simulink model "Q9_Simulink"  (R2019a)
settings: Solver=VariableStepAuto  StartTime=0.0  StopTime=simTime  RelTol=1e-8
values from neighbouring files (symbols this model uses):
  atan_scale = 100    [Q6.mat]    (also in Q8.mat)
  b_1 = 0.0029    [Q6.mat]    (also in Q8.mat)
  b_2 = 0.0002    [Q6.mat]    (also in Q8.mat)
  b_3 = 0.00015    [Q6.mat]    (also in Q8.mat)
  C = [1 0 0 0 0 0 0 1 0 0 0 0 ... (18 elements, 3x6)]    [Q6.mat]    (also in Q8.mat)
  C_ref = [1.22433209487 0.111020135599 0.137798657392 0.044869064232 0.221712033644 0.0486858100967]    [Q8.mat]
  F = [0.991402974605 -4.28040333336 0.0119339997062 5.93452176144 2.30402133564e-05 0.0230057113747 0.0039792647266 0.986787027522 1.59283068262e-05 0.0119155228703 1.84337564103e-08 2.30188301989e-05 ... (36 elements, 6x6)]    [Q8.mat]
  f_m = 0.00325471482319    [Q6.mat]
  f_m_time = 5    [Q6.mat]
  G = [0.00319046326914 1.59170589064 6.37978954487e-06 0.00637132273049 4.91886463074e-09 7.3735025641e-06]    [Q8.mat]
  h_sol = 17.717102911    [Q6.mat]
  J_1 = 0.0025    [Q6.mat]    (also in Q8.mat)
  J_2 = 0.0018    [Q6.mat]    (also in Q8.mat)
  J_3 = 0.0018    [Q6.mat]    (also in Q8.mat)
  k_1 = 2.7    [Q6.mat]    (also in Q8.mat)
  k_2 = 2.6    [Q6.mat]    (also in Q8.mat)
  Kc = [0.596249461469 0.0540667816687 0.0671079159043 0.0218512244326 0.10797371172 0.0237099788309]    [Q8.mat]
  mu_0 = 0    [Q6.mat]
  mu_1_sol = -0.0172499885629    [Q6.mat]
  T_Cm = 0.0969711017207    [Q6.mat]    (also in Q8.mat)
  T_Cp = 0.0714454263135    [Q6.mat]    (also in Q8.mat)
  T_s = 0.004    [Q6.mat]
  theta_3_ref = 1.57079632679    [Q8.mat]
  Ts = 0.004    [Q8.mat]
  var_r0 = 0.0043741038014    [Q6.mat]
  w_th = 0.75    [Q6.mat]    (also in Q8.mat)
  x_0 = [0 0 0 0 0 0]    [Q6.mat]
undefined symbols (not defined in the file or in its folder): C_f, C_V_d, G_V, G_y1_d, G_y2_d, G_y3_d, L_d, L_V_d, P_V_d, sigma_meas
settings Model: Creator=dimpa  LastModifiedBy=Ian
settings DataIOCC: ReturnWorkspaceOutputs=off
settings DebuggingCC: ArithmeticOperatorsInVariantConditions=warning
settings SFSimCC: SimUseLocalCustomCode=off
settings RTWCC: RTWUseLocalCustomCode=off

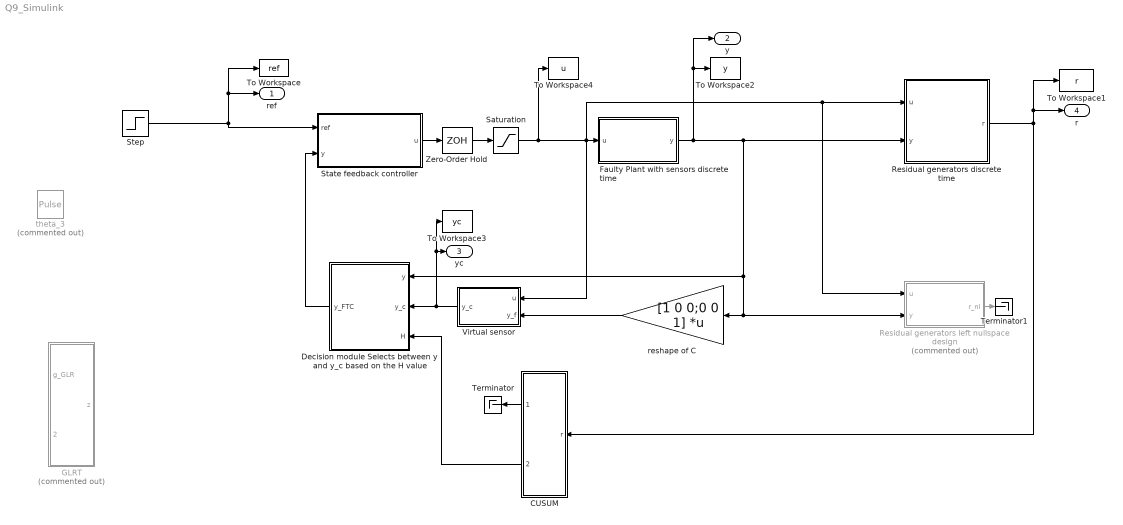
== system Q9_Simulink ==
  CUSUM : Subsystem
  Decision module Selects between y and y_c based on the H value : Subsystem
  Faulty Plant with sensors discrete time : Subsystem
  GLRT : Subsystem  Commented=on
  Residual generators discrete time : Subsystem
  Residual generators left nullspace design : Subsystem  Commented=on
  Saturation : Saturate  UpperLimit=2  LowerLimit=-2
  State feedback controller : Subsystem
  Step : Step  Time=15  After=theta_3_ref  SampleTime=0
  Terminator : Terminator
  Terminator1 : Terminator
  To Workspace : ToWorkspace  VariableName=ref  SaveFormat=Structure With Time  SampleTime=-1
  To Workspace1 : ToWorkspace  VariableName=r  SaveFormat=Structure With Time  SampleTime=-1
  To Workspace2 : ToWorkspace  VariableName=y  SaveFormat=Structure With Time  SampleTime=-1
  To Workspace3 : ToWorkspace  VariableName=yc  SaveFormat=Structure With Time  SampleTime=-1
  To Workspace4 : ToWorkspace  VariableName=u  SaveFormat=Structure With Time  SampleTime=-1
  Virtual sensor : Subsystem
  Zero-Order Hold : ZeroOrderHold  SampleTime=T_s
  reshape of C : Gain  Gain=[1 0 0;0 0 1]  Multiplication=Matrix(K*u) (u vector)
  theta_3 : DiscretePulseGenerator  Commented=on  PulseType=Time based  Amplitude=theta_3_ref  Period=30  PulseWidth=50
  ref : Outport  VectorParamsAs1DForOutWhenUnconnected=on
  y : Outport  Port=2  VectorParamsAs1DForOutWhenUnconnected=on
  yc : Outport  Port=3  VectorParamsAs1DForOutWhenUnconnected=on
  r : Outport  Port=4  VectorParamsAs1DForOutWhenUnconnected=on
  wires:
  State feedback controller/1(u) -> Zero-Order Hold/1
  Saturation/1 -> To Workspace4/1, Virtual sensor/1(u), Residual generators discrete time/1(u), Residual generators left nullspace design/1(u), Faulty Plant with sensors discrete time/1(u)
  Faulty Plant with sensors discrete time/1(y) -> y/1, To Workspace2/1, Residual generators discrete time/2(y), Decision module Selects between y and y_c based on the H value/1(y), reshape of C/1, Residual generators left nullspace design/2(y)
  Step/1 -> State feedback controller/1(ref), ref/1, To Workspace/1
  Virtual sensor/1(y_c) -> yc/1, To Workspace3/1, Decision module Selects between y and y_c based on the H value/2(y_c)
  reshape of C/1 -> Virtual sensor/2(y_f)
  Zero-Order Hold/1 -> Saturation/1
  CUSUM/2(H_CUSUM) -> Decision module Selects between y and y_c based on the H value/3(H)
  CUSUM/1(g_CUSUM) -> Terminator/1
  Residual generators left nullspace design/1(r_nl) -> Terminator1/1
  Residual generators discrete time/1(r) -> r/1, To Workspace1/1, CUSUM/1(r)
  Decision module Selects between y and y_c based on the H value/1(y_FTC) -> State feedback controller/2(y)

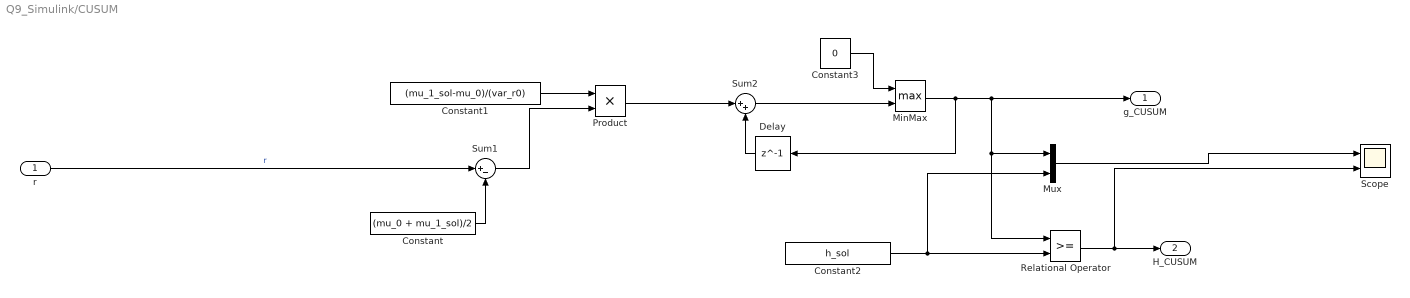
== system Q9_Simulink/CUSUM ==
  r : Inport
  Constant : Constant  Value=(mu_0 + mu_1_sol)/2
  Constant1 : Constant  Value=(mu_1_sol-mu_0)/(var_r0)
  Constant2 : Constant  Value=h_sol  VectorParams1D=off
  Constant3 : Constant  Value=0
  Delay : Delay  DelayLength=1  SampleTime=0.004
  MinMax : MinMax  Function=max  Inputs=2
  Mux : Mux  Inputs=2
  Product : Product
  Relational Operator : RelationalOperator  OutDataTypeStr=boolean  RndMeth=Simplest
  Scope : Scope  NumInputPorts=2
  Sum1 : Sum  Inputs=|+-
  Sum2 : Sum  Inputs=|++
  g_CUSUM : Outport
  H_CUSUM : Outport  Port=2
  wires:
  MinMax/1 -> Delay/1, g_CUSUM/1, Mux/1, Relational Operator/1
  Mux/1 -> Scope/1
  Delay/1 -> Sum2/2
  Constant2/1 -> Mux/2, Relational Operator/2
  Product/1 -> Sum2/1
  Constant3/1 -> MinMax/1
  Constant/1 -> Sum1/2
  Constant1/1 -> Product/1
  Sum1/1 -> Product/2
  Relational Operator/1 -> H_CUSUM/1, Scope/2
  Sum2/1 -> MinMax/2
  r/1 -> Sum1/1  "r"

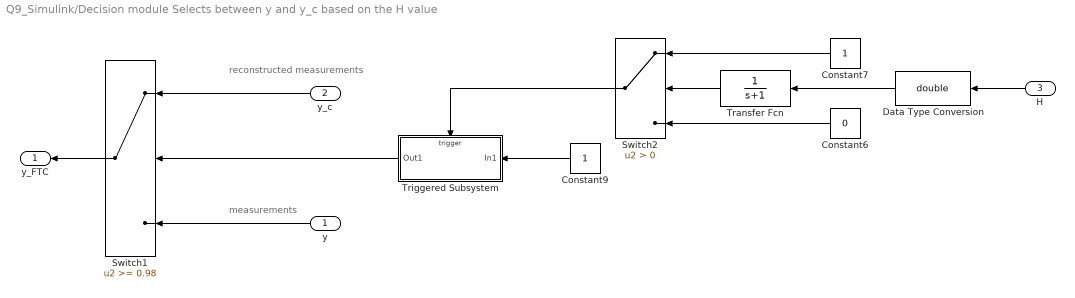
== system Q9_Simulink/Decision module Selects between y and y_c based on the H value ==
  note: measurements
  note: reconstructed
      | measurements
  y : Inport
  y_c : Inport  Port=2
  H : Inport  Port=3
  Constant6 : Constant  Value=0
  Constant7 : Constant
  Constant9 : Constant
  Data Type Conversion : DataTypeConversion  OutDataTypeStr=double
  Switch1 : Switch  Threshold=0.98
  Switch2 : Switch  Criteria=u2 > Threshold
  Transfer Fcn : TransferFcn  Denominator=[1 1]
  Triggered Subsystem : Subsystem  TreatAsAtomicUnit=on
  y_FTC : Outport
  wires:
  Switch1/1 -> y_FTC/1
  Constant6/1 -> Switch2/3
  Constant9/1 -> Triggered Subsystem/1(In1)
  Switch2/1 -> Triggered Subsystem/Trigger
  Constant7/1 -> Switch2/1
  Transfer Fcn/1 -> Switch2/2
  y/1 -> Switch1/3
  y_c/1 -> Switch1/1
  H/1 -> Data Type Conversion/1
  Triggered Subsystem/1(Out1) -> Switch1/2
  Data Type Conversion/1 -> Transfer Fcn/1

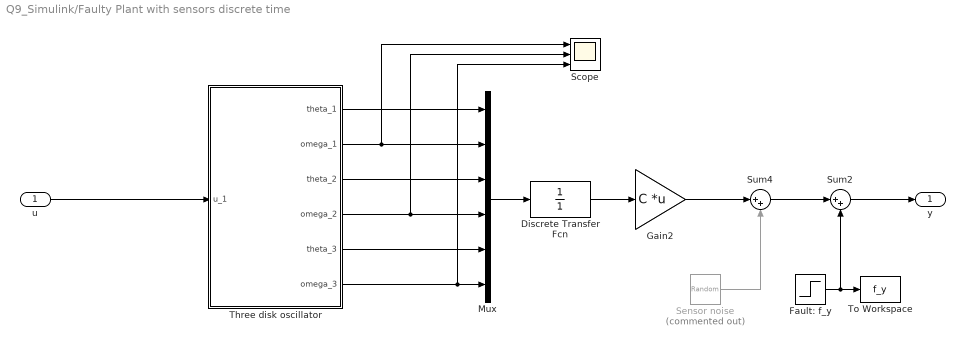
== system Q9_Simulink/Faulty Plant with sensors discrete time ==
  u : Inport
  Discrete Transfer Fcn : DiscreteTransferFcn  Denominator=[1]  SampleTime=T_s
  Fault: f_y : Step  Time=f_m_time  Before=[0;0;0]  After=f_m  SampleTime=0
  Gain2 : Gain  Gain=C  Multiplication=Matrix(K*u) (u vector)
  Mux : Mux  Inputs=6
  Scope : Scope  NumInputPorts=3
  Sensor noise : RandomNumber  Commented=on  Mean=zeros(3,1)  Variance=sigma_meas  SampleTime=T_s
  Sum2 : Sum  Inputs=|++
  Sum4 : Sum  Inputs=|++
  Three disk oscillator : Subsystem
  To Workspace : ToWorkspace  VariableName=f_y  SaveFormat=Structure With Time  SampleTime=-1
  y : Outport
  wires:
  u/1 -> Three disk oscillator/1(u_1)
  Three disk oscillator/2(omega_1) -> Scope/1, Mux/2
  Three disk oscillator/1(theta_1) -> Mux/1
  Mux/1 -> Discrete Transfer Fcn/1
  Three disk oscillator/4(omega_2) -> Scope/2, Mux/4
  Three disk oscillator/3(theta_2) -> Mux/3
  Discrete Transfer Fcn/1 -> Gain2/1
  Gain2/1 -> Sum4/1
  Sum2/1 -> y/1
  Sensor noise/1 -> Sum4/2
  Three disk oscillator/6(omega_3) -> Scope/3, Mux/6
  Three disk oscillator/5(theta_3) -> Mux/5
  Sum4/1 -> Sum2/1
  Fault: f_y/1 -> To Workspace/1, Sum2/2

== system Q9_Simulink/GLRT ==
  z : Inport
  g_GLR : Outport
  H_GLR : Outport  Port=2

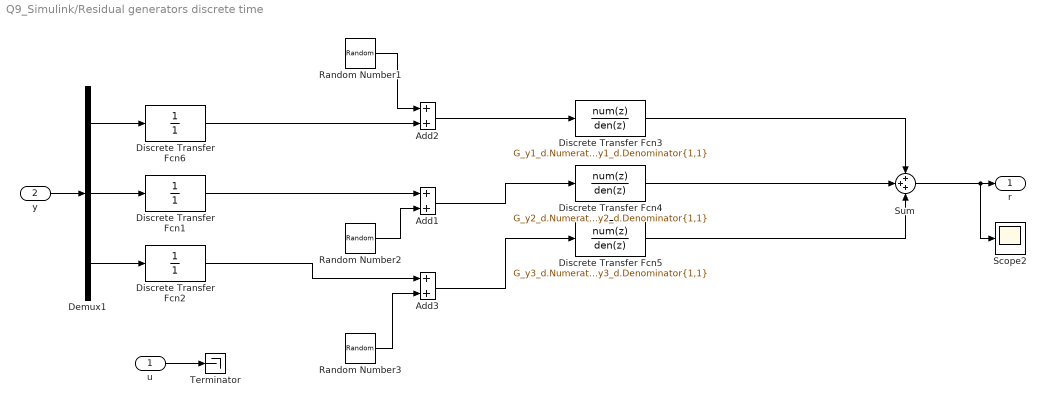
== system Q9_Simulink/Residual generators discrete time ==
  u : Inport
  y : Inport  Port=2
  Add1 : Sum
  Add2 : Sum
  Add3 : Sum
  Demux1 : Demux  Outputs=3
  Discrete Transfer Fcn1 : DiscreteTransferFcn  Denominator=[1]  SampleTime=0.004
  Discrete Transfer Fcn2 : DiscreteTransferFcn  Denominator=[1]  SampleTime=0.004
  Discrete Transfer Fcn3 : DiscreteTransferFcn  Numerator=G_y1_d.Numerator{1,1}  Denominator=G_y1_d.Denominator{1,1}
  Discrete Transfer Fcn4 : DiscreteTransferFcn  Numerator=G_y2_d.Numerator{1,1}  Denominator=G_y2_d.Denominator{1,1}
  Discrete Transfer Fcn5 : DiscreteTransferFcn  Numerator=G_y3_d.Numerator{1,1}  Denominator=G_y3_d.Denominator{1,1}
  Discrete Transfer Fcn6 : DiscreteTransferFcn  Denominator=[1]  SampleTime=0.004
  Random Number1 : RandomNumber  Variance=0.01^2  Seed=124234  SampleTime=T_s
  Random Number2 : RandomNumber  Variance=0.01^2  Seed=245364  SampleTime=T_s
  Random Number3 : RandomNumber  Variance=0.01^2  Seed=1465  SampleTime=T_s
  Scope2 : Scope
  Sum : Sum  Inputs=+++
  Terminator : Terminator
  r : Outport
  wires:
  u/1 -> Terminator/1
  Discrete Transfer Fcn4/1 -> Sum/2
  Sum/1 -> r/1, Scope2/1
  Add1/1 -> Discrete Transfer Fcn4/1
  Discrete Transfer Fcn5/1 -> Sum/3
  Random Number2/1 -> Add1/2
  Discrete Transfer Fcn3/1 -> Sum/1
  Random Number3/1 -> Add3/2
  Discrete Transfer Fcn2/1 -> Add3/1
  Add3/1 -> Discrete Transfer Fcn5/1
  y/1 -> Demux1/1
  Demux1/1 -> Discrete Transfer Fcn6/1
  Discrete Transfer Fcn6/1 -> Add2/2
  Random Number1/1 -> Add2/1
  Add2/1 -> Discrete Transfer Fcn3/1
  Demux1/2 -> Discrete Transfer Fcn1/1
  Discrete Transfer Fcn1/1 -> Add1/1
  Demux1/3 -> Discrete Transfer Fcn2/1

== system Q9_Simulink/Residual generators left nullspace design ==
  u : Inport
  y : Inport  Port=2
  r_nl : Outport

== system Q9_Simulink/State feedback controller ==
  ref : Inport
  y : Inport  Port=2
  State feedback with linear observer : Subsystem
  u : Outport
  wires:
  ref/1 -> State feedback with linear observer/1(ref)
  y/1 -> State feedback with linear observer/2(y)
  State feedback with linear observer/1(u) -> u/1

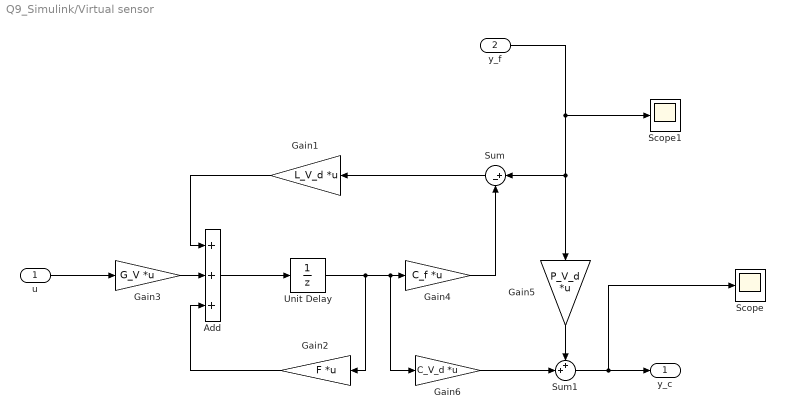
== system Q9_Simulink/Virtual sensor ==
  u : Inport
  y_f : Inport  Port=2
  Add : Sum  Inputs=+++
  Gain1 : Gain  Gain=L_V_d  Multiplication=Matrix(K*u)
  Gain2 : Gain  Gain=F  Multiplication=Matrix(K*u)
  Gain3 : Gain  Gain=G_V  Multiplication=Matrix(K*u)
  Gain4 : Gain  Gain=C_f  Multiplication=Matrix(K*u)
  Gain5 : Gain  Gain=P_V_d  Multiplication=Matrix(K*u)
  Gain6 : Gain  Gain=C_V_d  Multiplication=Matrix(K*u)
  Scope : Scope
  Scope1 : Scope
  Sum : Sum  Inputs=|+-
  Sum1 : Sum  Inputs=++|
  Unit Delay : UnitDelay  SampleTime=Ts  HasFrameUpgradeWarning=on
  y_c : Outport
  wires:
  u/1 -> Gain3/1
  Gain3/1 -> Add/2
  Gain1/1 -> Add/1
  Gain2/1 -> Add/3
  Add/1 -> Unit Delay/1
  Unit Delay/1 -> Gain6/1, Gain4/1, Gain2/1
  Sum/1 -> Gain1/1
  Gain4/1 -> Sum/2
  y_f/1 -> Scope1/1, Sum/1, Gain5/1
  Gain6/1 -> Sum1/2
  Gain5/1 -> Sum1/1
  Sum1/1 -> Scope/1, y_c/1

== system Q9_Simulink/Decision module Selects between y and y_c based on the H value/Triggered Subsystem ==
  In1 : Inport
  Trigger : TriggerPort  VariantControl=Variant
  Out1 : Outport
  wires:
  In1/1 -> Out1/1

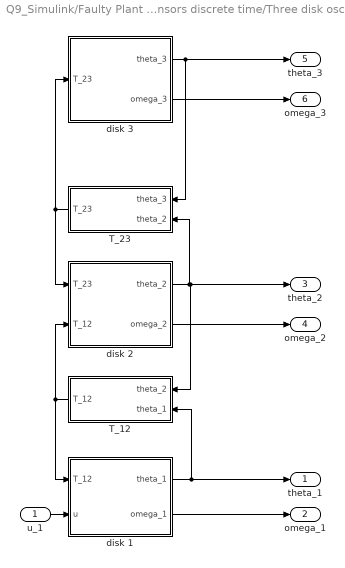
== system Q9_Simulink/Faulty Plant with sensors discrete time/Three disk oscillator ==
  u_1 : Inport
  T_12 : Subsystem
  T_23 : Subsystem
  disk 1 : Subsystem
  disk 2 : Subsystem
  disk 3 : Subsystem
  theta_1 : Outport
  omega_1 : Outport  Port=2
  theta_2 : Outport  Port=3
  omega_2 : Outport  Port=4
  theta_3 : Outport  Port=5
  omega_3 : Outport  Port=6
  wires:
  T_23/1(T_23) -> disk 2/1(T_23), disk 3/1(T_23)
  disk 1/1(theta_1) -> T_12/2(theta_1), theta_1/1
  disk 2/1(theta_2) -> T_23/2(theta_2), theta_2/1, T_12/1(theta_2)
  T_12/1(T_12) -> disk 1/1(T_12), disk 2/2(T_12)
  disk 3/2(omega_3) -> omega_3/1
  disk 1/2(omega_1) -> omega_1/1
  disk 2/2(omega_2) -> omega_2/1
  u_1/1 -> disk 1/2(u)
  disk 3/1(theta_3) -> theta_3/1, T_23/1(theta_3)

== system Q9_Simulink/State feedback controller/State feedback with linear observer ==
  ref : Inport
  y : Inport  Port=2
  State observer with integral action : Subsystem
  State-feedback : Subsystem
  u : Outport
  wires:
  State observer with integral action/1(x_hat) -> State-feedback/2(x_hat)
  y/1 -> State observer with integral action/2(y)
  ref/1 -> State-feedback/1(ref)
  State-feedback/1(u) -> u/1, State observer with integral action/1(u)

== system Q9_Simulink/Faulty Plant with sensors discrete time/Three disk oscillator/T_12 ==
  theta_2 : Inport
  theta_1 : Inport  Port=2
  Gain : Gain  Gain=k_1
  Sum : Sum  Inputs=|+-
  T_12 : Outport
  wires:
  theta_2/1 -> Sum/2
  theta_1/1 -> Sum/1
  Sum/1 -> Gain/1
  Gain/1 -> T_12/1

== system Q9_Simulink/Faulty Plant with sensors discrete time/Three disk oscillator/T_23 ==
  theta_3 : Inport
  theta_2 : Inport  Port=2
  Gain : Gain  Gain=k_2
  Sum : Sum  Inputs=-+|
  T_23 : Outport
  wires:
  Gain/1 -> T_23/1
  Sum/1 -> Gain/1
  theta_3/1 -> Sum/1
  theta_2/1 -> Sum/2

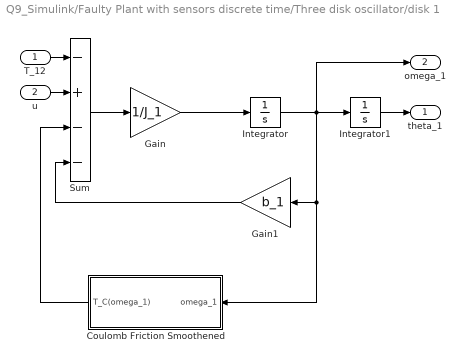
== system Q9_Simulink/Faulty Plant with sensors discrete time/Three disk oscillator/disk 1 ==
  T_12 : Inport
  u : Inport  Port=2
  Coulomb Friction Smoothened : Subsystem
  Gain : Gain  Gain=1/J_1
  Gain1 : Gain  Gain=b_1
  Integrator : Integrator  InitialCondition=x_0(2)
  Integrator1 : Integrator  InitialCondition=x_0(1)
  Sum : Sum  Inputs=-+--
  theta_1 : Outport
  omega_1 : Outport  Port=2
  wires:
  Sum/1 -> Gain/1
  Integrator/1 -> Integrator1/1, omega_1/1, Coulomb Friction Smoothened/1(omega_1), Gain1/1
  Gain1/1 -> Sum/4
  Integrator1/1 -> theta_1/1
  T_12/1 -> Sum/1
  u/1 -> Sum/2
  Gain/1 -> Integrator/1
  Coulomb Friction Smoothened/1(T_C(omega_1)) -> Sum/3

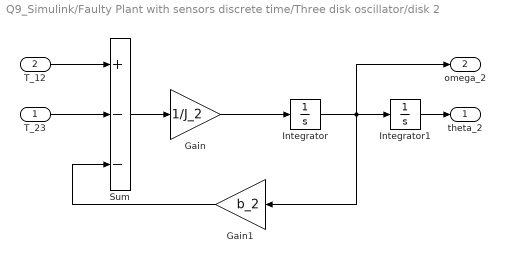
== system Q9_Simulink/Faulty Plant with sensors discrete time/Three disk oscillator/disk 2 ==
  T_23 : Inport
  T_12 : Inport  Port=2
  Gain : Gain  Gain=1/J_2
  Gain1 : Gain  Gain=b_2
  Integrator : Integrator  InitialCondition=x_0(4)
  Integrator1 : Integrator  InitialCondition=x_0(3)
  Sum : Sum  Inputs=+--
  theta_2 : Outport
  omega_2 : Outport  Port=2
  wires:
  T_23/1 -> Sum/2
  T_12/1 -> Sum/1
  Integrator1/1 -> theta_2/1
  Gain1/1 -> Sum/3
  Gain/1 -> Integrator/1
  Integrator/1 -> Integrator1/1, Gain1/1, omega_2/1
  Sum/1 -> Gain/1

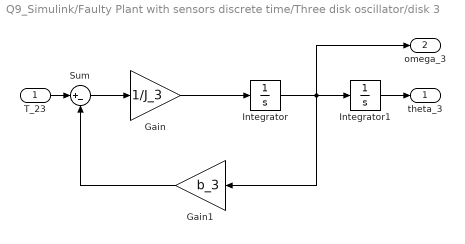
== system Q9_Simulink/Faulty Plant with sensors discrete time/Three disk oscillator/disk 3 ==
  T_23 : Inport
  Gain : Gain  Gain=1/J_3
  Gain1 : Gain  Gain=b_3
  Integrator : Integrator  InitialCondition=x_0(6)
  Integrator1 : Integrator  InitialCondition=x_0(5)
  Sum : Sum  Inputs=|+-
  theta_3 : Outport
  omega_3 : Outport  Port=2
  wires:
  Sum/1 -> Gain/1
  Integrator/1 -> Integrator1/1, omega_3/1, Gain1/1
  Gain/1 -> Integrator/1
  Gain1/1 -> Sum/2
  Integrator1/1 -> theta_3/1
  T_23/1 -> Sum/1

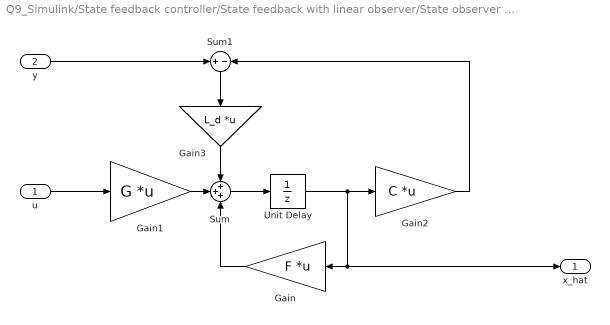
== system Q9_Simulink/State feedback controller/State feedback with linear observer/State observer with integral action ==
  u : Inport
  y : Inport  Port=2
  Gain : Gain  Gain=F  Multiplication=Matrix(K*u) (u vector)
  Gain1 : Gain  Gain=G  Multiplication=Matrix(K*u) (u vector)
  Gain2 : Gain  Gain=C  Multiplication=Matrix(K*u) (u vector)
  Gain3 : Gain  Gain=L_d  Multiplication=Matrix(K*u) (u vector)
  Sum : Sum  Inputs=+++
  Sum1 : Sum  Inputs=+-
  Unit Delay : UnitDelay  SampleTime=T_s  HasFrameUpgradeWarning=on
  x_hat : Outport
  wires:
  y/1 -> Sum1/1
  Sum1/1 -> Gain3/1
  Sum/1 -> Unit Delay/1
  Gain2/1 -> Sum1/2
  u/1 -> Gain1/1
  Gain1/1 -> Sum/2
  Gain/1 -> Sum/3
  Gain3/1 -> Sum/1
  Unit Delay/1 -> x_hat/1, Gain/1, Gain2/1

== system Q9_Simulink/State feedback controller/State feedback with linear observer/State-feedback ==
  ref : Inport
  x_hat : Inport  Port=2
  Gain : Gain  Gain=Kc  Multiplication=Matrix(K*u) (u vector)
  Gain1 : Gain  Gain=C_ref  Multiplication=Matrix(K*u) (u vector)
  Sum1 : Sum  Inputs=|+-
  u : Outport
  wires:
  Gain1/1 -> Sum1/1
  Sum1/1 -> Gain/1
  x_hat/1 -> Sum1/2
  Gain/1 -> u/1
  ref/1 -> Gain1/1

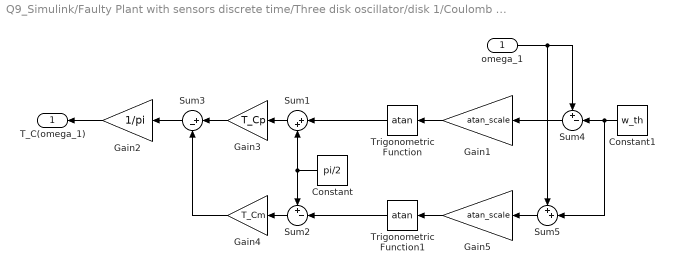
== system Q9_Simulink/Faulty Plant with sensors discrete time/Three disk oscillator/disk 1/Coulomb Friction Smoothened ==
  omega_1 : Inport
  Constant : Constant  Value=pi/2
  Constant1 : Constant  Value=w_th
  Gain1 : Gain  Gain=atan_scale
  Gain2 : Gain  Gain=1/pi
  Gain3 : Gain  Gain=T_Cp
  Gain4 : Gain  Gain=T_Cm
  Gain5 : Gain  Gain=atan_scale
  Sum1 : Sum  Inputs=|++
  Sum2 : Sum  Inputs=+-|
  Sum3 : Sum  Inputs=|+-
  Sum4 : Sum  Inputs=+-|
  Sum5 : Sum  Inputs=++|
  Trigonometric Function : Trigonometry  Operator=atan
  Trigonometric Function1 : Trigonometry  Operator=atan
  T_C(omega_1) : Outport
  wires:
  Gain1/1 -> Trigonometric Function/1
  Sum1/1 -> Gain3/1
  Constant/1 -> Sum2/1, Sum1/2
  Sum2/1 -> Gain4/1
  Sum3/1 -> Gain2/1
  Trigonometric Function/1 -> Sum1/1
  Gain4/1 -> Sum3/2
  Gain2/1 -> T_C(omega_1)/1
  omega_1/1 -> Sum5/1, Sum4/1
  Gain3/1 -> Sum3/1
  Sum4/1 -> Gain1/1
  Constant1/1 -> Sum5/2, Sum4/2
  Gain5/1 -> Trigonometric Function1/1
  Sum5/1 -> Gain5/1
  Trigonometric Function1/1 -> Sum2/2
